simulink model "quad_control_2attached"  (R2016a)
settings: Solver=FixedStepAuto  StartTime=0.0  StopTime=60  FixedStep=0.025  RelTol=1e-3
InitFcn:
  | global clientID;
  | clientID=-1;
values from neighbouring files (symbols this model uses):
  X = reshape(X, size(A_t))    [RiccatiCov.m]
undefined symbols (not defined in the file or in its folder): Y, Z
libraries: robotlib x5, dspindex x2
settings Model: Creator=Kleber Cabral  LastModifiedBy=Kleber Cabral
settings DataIOCC: SaveFormat=Array
settings DebuggingCC: SolverPrmCheckMsg=warning
settings HardwareCC: ProdBitPerPointer=32  ProdLargestAtomicFloat=None  ProdIntDivRoundTo=Undefined  ProdEndianess=Unspecified  ProdWordSize=32  ProdHWDeviceType=32-bit Generic
settings ModelReferenceCC: PropagateSignalLabelsOutOfModel=off
settings ConfigComp: CovModelRefEnable=Off  CovSFcnEnable=off

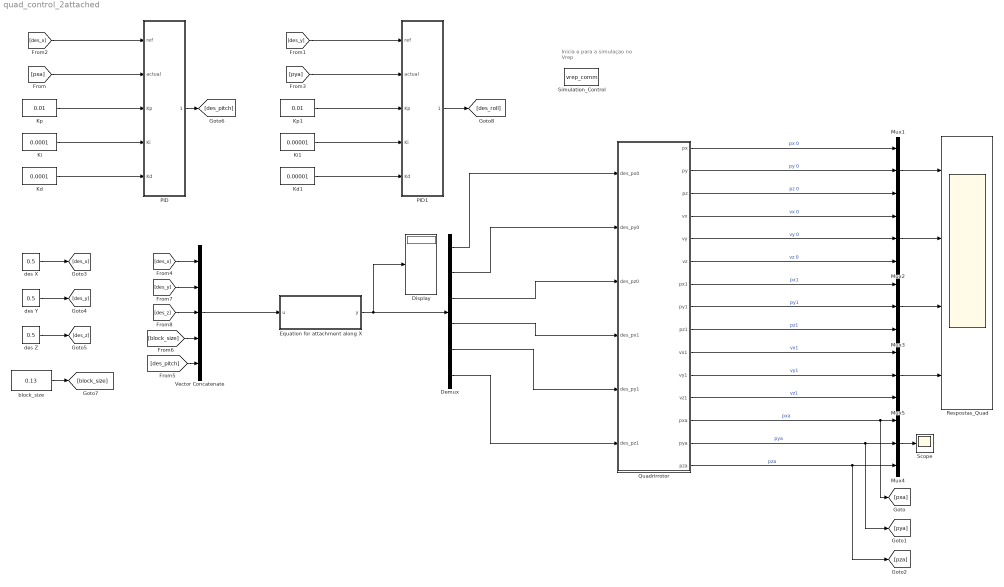
== system quad_control_2attached ==
  note: Inicia e para a simulaçao no Vrep
  Demux : Demux  Outputs=6
  Display : Display
      settings: Decimation=3
  Equation for attachment along X : MATLAB Function  TreatAsAtomicUnit=on
  Kd : Constant  Value=0.0001
  Kd1 : Constant  Value=0.00001
  Ki : Constant  Value=0.0001
  Ki1 : Constant  Value=0.00001
  Kp : Constant  Value=0.01
  Kp1 : Constant  Value=0.01
  Mux{1..5} (5 alike) : Mux  Inputs=3
  PID : Subsystem
  PID1 : Subsystem
  Quadrirrotor : Subsystem
  Respostas_Quad : Scope  NumInputPorts=4
  Scope : Scope
  Simulation_Control : S-Function  FunctionName=vrep_comm  SFunctionDeploymentMode=off  EnableBusSupport=off
  Vector Concatenate : Concatenate  NumInputs=5
  block_size : Constant  Value=0.13
  des X : Constant  Value=0.5
  des Y : Constant  Value=0.5
  des Z : Constant  Value=0.5
  wires:
  Mux1/1 -> Respostas_Quad/1
  Mux2/1 -> Respostas_Quad/2
  Quadrirrotor/1(px) -> Mux1/1  "px 0"
  Quadrirrotor/3(pz) -> Mux1/3  "pz 0"
  Quadrirrotor/2(py) -> Mux1/2  "py 0"
  Quadrirrotor/5(vy) -> Mux2/2  "vy 0"
  Quadrirrotor/4(vx) -> Mux2/1  "vx 0"
  Quadrirrotor/6(vz) -> Mux2/3  "vz 0"
  Mux3/1 -> Respostas_Quad/3
  Mux4/1 -> Scope/1
  Quadrirrotor/7(px1) -> Mux3/1  "px1"
  Quadrirrotor/8(py1) -> Mux3/2  "py1"
  Quadrirrotor/9(pz1) -> Mux3/3  "pz1"
  Mux5/1 -> Respostas_Quad/4
  Quadrirrotor/12(vz1) -> Mux5/3  "vz1"
  Quadrirrotor/11(vy1) -> Mux5/2  "vy1"
  Quadrirrotor/10(vx1) -> Mux5/1  "vx1"
  Quadrirrotor/13(pxa) -> [pxa], Mux4/1  "pxa"
  Quadrirrotor/15(pza) -> [pza], Mux4/3  "pza"
  Quadrirrotor/14(pya) -> [pya], Mux4/2  "pya"
  Kp/1 -> PID/3(Kp)
  Ki/1 -> PID/4(Ki)
  Kd/1 -> PID/5(Kd)
  [pxa] -> PID/2(actual)
  Kp1/1 -> PID1/3(Kp)
  Ki1/1 -> PID1/4(Ki)
  Kd1/1 -> PID1/5(Kd)
  [pya] -> PID1/2(actual)
  des X/1 -> [des_x]
  des Y/1 -> [des_y]
  des Z/1 -> [des_z]
  [des_x] -> PID/1(ref)
  [des_y] -> PID1/1(ref)
  PID/1(PID_out) -> [des_pitch]
  block_size/1 -> [block_size]
  [des_pitch] -> Vector Concatenate/5
  [block_size] -> Vector Concatenate/4
  Vector Concatenate/1 -> Equation for attachment along X/1(u)
  [des_x] -> Vector Concatenate/1
  [des_y] -> Vector Concatenate/2
  [des_z] -> Vector Concatenate/3
  PID1/1(PID_out) -> [des_roll]
  Demux/4 -> Quadrirrotor/4(des_px1)
  Demux/3 -> Quadrirrotor/3(des_pz0)
  Demux/5 -> Quadrirrotor/5(des_py1)
  Demux/2 -> Quadrirrotor/2(des_py0)
  Demux/6 -> Quadrirrotor/6(des_pz1)
  Demux/1 -> Quadrirrotor/1(des_px0)
  Equation for attachment along X/1(y) -> Display/1, Demux/1

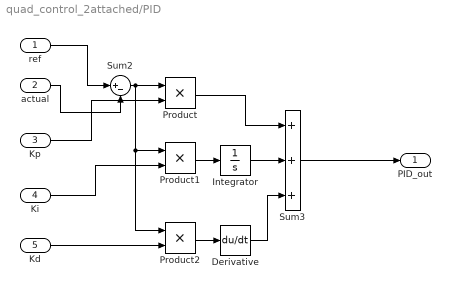
== system quad_control_2attached/PID ==
  ref : Inport
  actual : Inport  Port=2
  Kp : Inport  Port=3
  Ki : Inport  Port=4
  Kd : Inport  Port=5
  Derivative : Derivative
  Integrator : Integrator
  Product : Product
  Product1 : Product
  Product2 : Product
  Sum2 : Sum  Inputs=|+-
  Sum3 : Sum  Inputs=+++
  PID_out : Outport
  wires:
  Kd/1 -> Product2/2
  Integrator/1 -> Sum3/2
  Product2/1 -> Derivative/1
  Sum2/1 -> Product/1, Product2/1, Product1/1
  Product/1 -> Sum3/1
  actual/1 -> Sum2/2
  Kp/1 -> Product/2
  Sum3/1 -> PID_out/1
  Ki/1 -> Product1/2
  Product1/1 -> Integrator/1
  ref/1 -> Sum2/1
  Derivative/1 -> Sum3/3

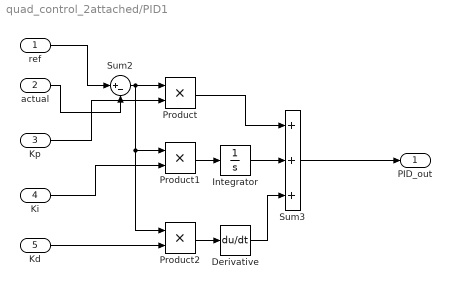
== system quad_control_2attached/PID1 ==
  ref : Inport
  actual : Inport  Port=2
  Kp : Inport  Port=3
  Ki : Inport  Port=4
  Kd : Inport  Port=5
  Derivative : Derivative
  Integrator : Integrator
  Product : Product
  Product1 : Product
  Product2 : Product
  Sum2 : Sum  Inputs=|+-
  Sum3 : Sum  Inputs=+++
  PID_out : Outport
  wires:
  Derivative/1 -> Sum3/3
  ref/1 -> Sum2/1
  Product1/1 -> Integrator/1
  Ki/1 -> Product1/2
  Sum3/1 -> PID_out/1
  Kp/1 -> Product/2
  actual/1 -> Sum2/2
  Product/1 -> Sum3/1
  Sum2/1 -> Product1/1, Product2/1, Product/1
  Product2/1 -> Derivative/1
  Integrator/1 -> Sum3/2
  Kd/1 -> Product2/2

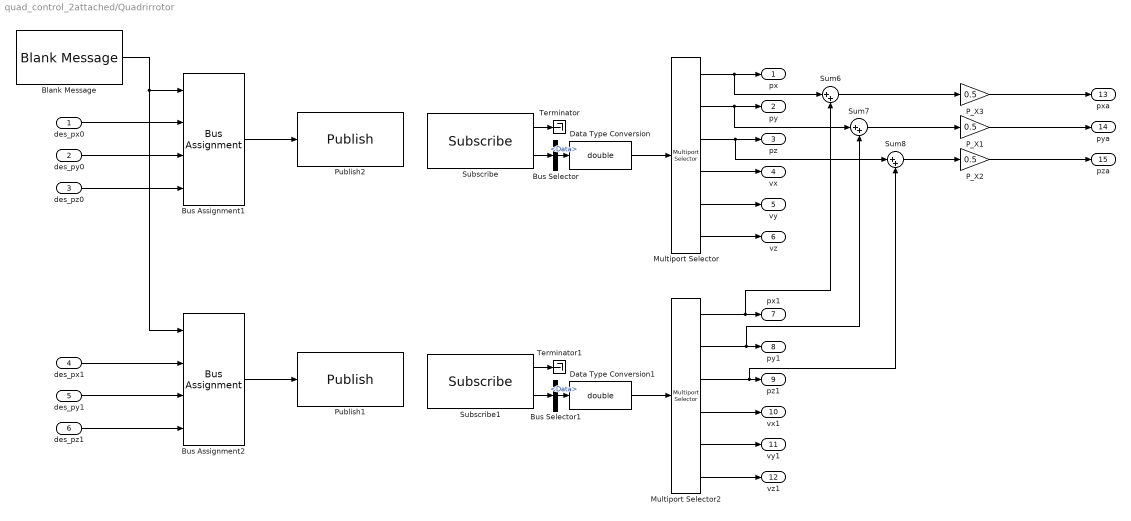
== system quad_control_2attached/Quadrirrotor ==
  des_px0 : Inport
  des_py0 : Inport  Port=2
  des_pz0 : Inport  Port=3
  des_px1 : Inport  Port=4
  des_py1 : Inport  Port=5
  des_pz1 : Inport  Port=6
  Blank Message : robotlib/Blank Message  SourceLibraryInfo=This block requires Robotics System Toolbox  messageType=geometry_msgs/Vector3  SampleTime=inf
  Bus Assignment1 : BusAssignment  DialogController=Simulink.DDGSource_BusAssignment  AssignedSignals=X,Y,Z
  Bus Assignment2 : BusAssignment  DialogController=Simulink.DDGSource_BusAssignment  AssignedSignals=X,Y,Z
  Bus Selector : BusSelector  OutputSignals=Data
  Bus Selector1 : BusSelector  OutputSignals=Data
  Data Type Conversion : DataTypeConversion  OutDataTypeStr=double
  Data Type Conversion1 : DataTypeConversion  OutDataTypeStr=double
  Multiport Selector : dspindex/Multiport Selector  rowsOrCols=Rows  idxCellArray={1,2,3,4,5,6}  idxErrMode=Clip Index
  Multiport Selector2 : dspindex/Multiport Selector  rowsOrCols=Rows  idxCellArray={1,2,3,4,5,6}  idxErrMode=Clip Index
  P_X1 : Gain  Gain=0.5
  P_X2 : Gain  Gain=0.5
  P_X3 : Gain  Gain=0.5
  Publish1 : robotlib/Publish  SourceLibraryInfo=This block requires Robotics System Toolbox  topicSource=Select from ROS network  topic=/desired_waypoint_1  messageType=geometry_msgs/Vector3  messageQueueLength=105
  Publish2 : robotlib/Publish  SourceLibraryInfo=This block requires Robotics System Toolbox  topicSource=Select from ROS network  topic=/desired_waypoint_0  messageType=geometry_msgs/Vector3  messageQueueLength=105
  Subscribe : robotlib/Subscribe  SourceLibraryInfo=This block requires Robotics System Toolbox  topicSource=Select from ROS network  topic=/quadrotor_states_0  messageType=std_msgs/Float32MultiArray  sampleTime=-1  messageQueueLength=51
  Subscribe1 : robotlib/Subscribe  SourceLibraryInfo=This block requires Robotics System Toolbox  topicSource=Select from ROS network  topic=/quadrotor_states_1  messageType=std_msgs/Float32MultiArray  sampleTime=-1  messageQueueLength=51
  Sum6 : Sum  Inputs=|++
  Sum7 : Sum  Inputs=|++
  Sum8 : Sum  Inputs=|++
  Terminator : Terminator
  Terminator1 : Terminator
  px : Outport
  py : Outport  Port=2
  pz : Outport  Port=3
  vx : Outport  Port=4
  vy : Outport  Port=5
  vz : Outport  Port=6
  px1 : Outport  Port=7
  py1 : Outport  Port=8
  pz1 : Outport  Port=9
  vx1 : Outport  Port=10
  vy1 : Outport  Port=11
  vz1 : Outport  Port=12
  pxa : Outport  Port=13
  pya : Outport  Port=14
  pza : Outport  Port=15
  wires:
  Multiport Selector/1 -> Sum6/1, px/1
  Multiport Selector/2 -> Sum7/1, py/1
  Multiport Selector/3 -> Sum8/1, pz/1
  Blank Message/1 -> Bus Assignment2/1, Bus Assignment1/1
  Subscribe/1 -> Terminator/1
  Subscribe/2 -> Bus Selector/1
  Data Type Conversion/1 -> Multiport Selector/1
  Multiport Selector/4 -> vx/1
  Multiport Selector/5 -> vy/1
  Multiport Selector/6 -> vz/1
  Bus Selector/1 -> Data Type Conversion/1  "<Data>"
  Bus Assignment1/1 -> Publish2/1
  Bus Assignment2/1 -> Publish1/1
  Subscribe1/1 -> Terminator1/1
  Subscribe1/2 -> Bus Selector1/1
  Data Type Conversion1/1 -> Multiport Selector2/1
  Bus Selector1/1 -> Data Type Conversion1/1  "<Data>"
  Sum6/1 -> P_X3/1
  Multiport Selector2/1 -> Sum6/2, px1/1
  Multiport Selector2/2 -> Sum7/2, py1/1
  Multiport Selector2/3 -> Sum8/2, pz1/1
  Multiport Selector2/4 -> vx1/1
  Multiport Selector2/5 -> vy1/1
  Multiport Selector2/6 -> vz1/1
  P_X3/1 -> pxa/1
  Sum7/1 -> P_X1/1
  Sum8/1 -> P_X2/1
  P_X2/1 -> pza/1
  des_py0/1 -> Bus Assignment1/3
  des_px0/1 -> Bus Assignment1/2
  des_pz0/1 -> Bus Assignment1/4
  P_X1/1 -> pya/1
  des_px1/1 -> Bus Assignment2/2
  des_py1/1 -> Bus Assignment2/3
  des_pz1/1 -> Bus Assignment2/4

== matlab function quad_control_2attached/Equation for attachment along X ==
  data: u input; y output
function y = fcn(u)
%#codegen
y=[eye(3);eye(3)]*[u(1);u(2);u(3)] + [-1;0;0;1;0;0]*(u(4)/2)+[0;0;1;0;0;-1]*u(5);
